simulink model "diagbloco"  (R2022a)
settings: Solver=FixedStepAuto  StartTime=0.0  StopTime=20  FixedStep=0.00001  MaxStep=0.0001  RelTol=1e-3
values from neighbouring files (symbols this model uses):
  K1 = [k1,k2 ... (first row only)    [WorkspaceK1_K2_K3.m]
  K2 = [k5,0 ... (first row only)    [WorkspaceK1_K2_K3.m]
  K3 = [k7 ... (first row only)    [WorkspaceK1_K2_K3.m]
  w = l_e / sqrt(B_B / (2 * g))    [WorkspaceK1_K2_K3.m]
  X0 = [0 ... (first row only)    [WorkspaceK1_K2_K3.m]
libraries: slpidlib x1
settings Model: Creator=Diogo Nazare  LastModifiedBy=Diogo Nazare

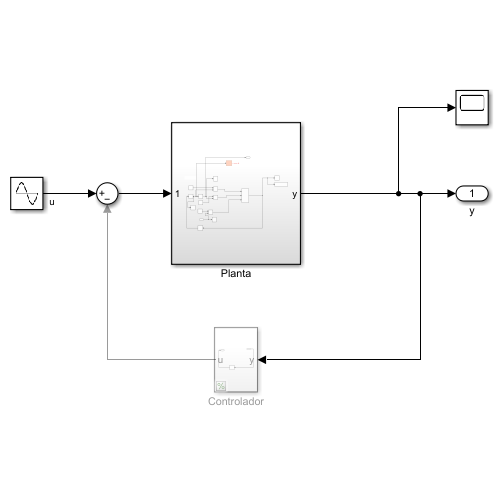
[thumbnail: Simulink's stored preview of the top-level diagram]
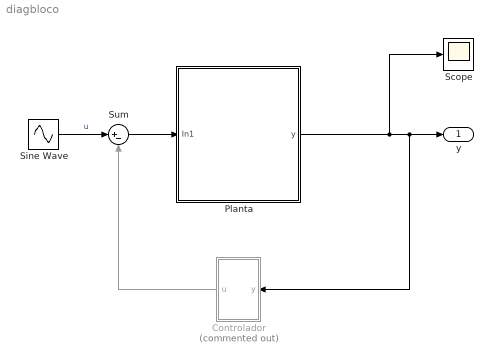
== system diagbloco ==
  Controlador : Subsystem  Commented=on
  Planta : Subsystem
  Scope : Scope
  Sine Wave : Sin  Frequency=w*2*pi  SampleTime=0
  Sum : Sum  Inputs=|+-
  y : Outport
  wires:
  Planta/1(y) -> Scope/1, Controlador/1(y), y/1
  Sine Wave/1 -> Sum/1  "u"
  Sum/1 -> Planta/1(In1)
  Controlador/1(u) -> Sum/2

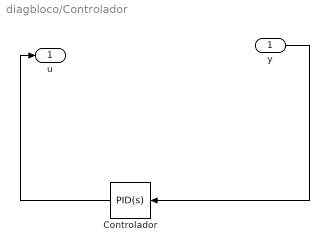
== system diagbloco/Controlador ==
  y : Inport
  Controlador : slpidlib/PID Controller  Controller=PID  Form=Parallel  TimeDomain=Continuous-time  UseExternalTs=off  SampleTime=-1  IntegratorMethod=Forward Euler  FilterMethod=Forward Euler  ControllerParametersSource=internal  P=1  I=1  UseKiTs=off  D=0  N=100  UseFilter=on  TunerSelectOption=Transfer Function Based (PID Tuner App)  InitialConditionSource=internal  InitialConditionForIntegrator=0  InitialConditionForFilter=0  DifferentiatorICPrevScaledInput=0  ExternalReset=none  TrackingMode=off  Kt=1  LimitOutput=off  SatLimitsSource=internal  UpperSaturationLimit=inf  LowerSaturationLimit=-inf  LinearizeAsGain=on  AntiWindupMode=none  Kb=1  POutMin=[]  POutMax=[]  IOutMin=[]  IOutMax=[]  DOutMin=[]  DOutMax=[]  NOutMin=[]  NOutMax=[]  SumOutMin=[]  SumOutMax=[]  SaturationOutMin=[]  SaturationOutMax=[]  PParamMin=[]  PParamMax=[]  IParamMin=[]  IParamMax=[]  DParamMin=[]  DParamMax=[]  NParamMin=[]  NParamMax=[]  KbParamMin=[]  KbParamMax=[]  KtParamMin=[]  KtParamMax=[]  KbOutMin=[]  KbOutMax=[]  KtOutMin=[]  KtOutMax=[]  IntegratorOutMin=[]  IntegratorOutMax=[]  FilterOutMin=[]  FilterOutMax=[]  SumI1OutMin=[]  SumI1OutMax=[]  SumI2OutMin=[]  SumI2OutMax=[]  SumI3OutMin=[]  SumI3OutMax=[]  SumI4OutMin=[]  SumI4OutMax=[]  SumDOutMin=[]  SumDOutMax=[]  DifferentiatorOutMin=[]  DifferentiatorOutMax=[]  FilterDiffOutCoefMin=[]  FilterDiffOutCoefMax=[]  ReciprocalOutMin=[]  ReciprocalOutMax=[]  SumDenOutMin=[]  SumDenOutMax=[]  SumNumOutMin=[]  SumNumOutMax=[]  DivideOutMin=[]  DivideOutMax=[]  UdiffTsProdOutMin=[]  UdiffTsProdOutMax=[]  NTsProdOutMin=[]  NTsProdOutMax=[]  UintegralTsProdOutMin=[]  UintegralTsProdOutMax=[]  UngainTsProdOutMin=[]  UngainTsProdOutMax=[]  IntegratorContinuousStateAttributes=''  IntegratorStateMustResolveToSignalObject=off  IntegratorRTWStateStorageClass=Auto  FilterContinuousStateAttributes=''  FilterStateMustResolveToSignalObject=off  FilterRTWStateStorageClass=Auto  ParallelPVariant=InternalParameters  IdealPVariant=Disabled  IVariant=InternalParameters  DVariant=InternalParameters  IntegratorVariant=Continuous  SatVariant=Disabled  AWVariant=Passthrough  PCopyVariant=Disabled  TRVariant=Disabled  FdbkBlocksVariant=Forward  IdealPFdbkVariant=Disabled  SatFdbkVariant=Disabled  DerivativeFilterVariant=ContFilter  NVariant=InternalParameters  NCopyVariant=Disabled  FilterICVariant=InternalICsFilter  IntegratorICVariant=InternalICs  ExternalResetVariant=Disabled  TRSumVariant=Passthrough  SumFdbkVariant=Disabled  SumVariant=Sum_PID  TsampFilterVariant=InternalTs  TsampNgainVariant=Passthrough  TsampIntegralVariant=Passthrough  ExternalSaturationOutDataTypeStr=Inherit: Same as second input  aMode=0
  u : Outport
  wires:
  y/1 -> Controlador/1
  Controlador/1 -> u/1

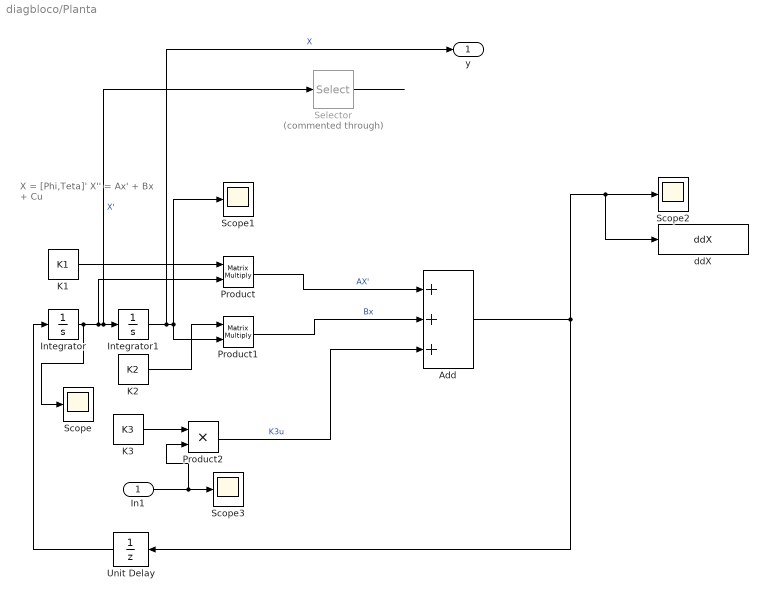
== system diagbloco/Planta ==
  note: X = [Phi,Teta]'
      | X'' = Ax' + Bx + Cu
  In1 : Inport
  Add : Sum  Inputs=+++
  Integrator : Integrator
  Integrator1 : Integrator
  K1 : Constant  Value=K1  VectorParams1D=off
  K2 : Constant  Value=K2  VectorParams1D=off
  K3 : Constant  Value=K3  VectorParams1D=off
  Product : Product  Multiplication=Matrix(*)
  Product1 : Product  Multiplication=Matrix(*)
  Product2 : Product
  Scope{,1..3} (4 alike) : Scope
  Selector : Selector  Commented=through  InputPortWidth=3  IndexOptions=Index vector (dialog)  Indices=[1 3]  OutputSizes=1
  Unit Delay : UnitDelay  InitialCondition=X0  SampleTime=-1  HasFrameUpgradeWarning=on
  ddX : ToWorkspace  VariableName=ddX  SampleTime=-1
  y : Outport
  wires:
  Add/1 -> Unit Delay/1, ddX/1, Scope2/1
  Product1/1 -> Add/2  "Bx"
  K1/1 -> Product/1
  K2/1 -> Product1/1
  Integrator1/1 -> y/1, Product1/2, Scope1/1  "X"
  Integrator/1 -> Scope/1, Selector/1, Integrator1/1, Product/2  "X'"
  Product/1 -> Add/1  "AX'"
  Unit Delay/1 -> Integrator/1
  K3/1 -> Product2/1
  Product2/1 -> Add/3  "K3u"
  In1/1 -> Product2/2, Scope3/1
  Selector/1 -> ?
